simulink model "Strife_Simulation"  (R2020b)
settings: Solver=VariableStepAuto  StartTime=0.0  StopTime=10.0  RelTol=1e-3
libraries: simulink_extras x1, shared3dof x1
settings Model: Creator=bowen  LastModifiedBy=bowen

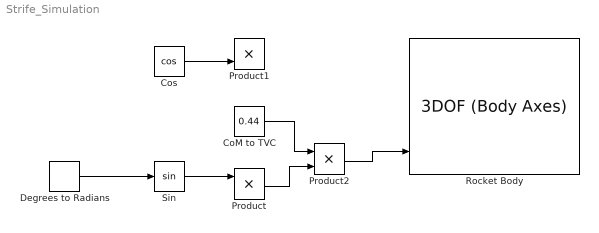
== system Strife_Simulation ==
  CoM to TVC : Constant  Value=0.44
  Cos : Trigonometry  Operator=cos
  Degrees to Radians : simulink_extras/Transformations/Degrees to Radians
  Product : Product
  Product1 : Product
  Product2 : Product
  Rocket Body : shared3dof/3DOF (Body Axes)  units=Metric (MKS)  mtype=Fixed  v_ini=100  theta_ini=0  alpha_ini=0  pos_ini=[0 0]  q_ini=0  mass=1.0  mass_e=0.5  mass_f=3.0  Iyy=1.0  Iyy_e=0.5  Iyy_f=3.0  g_in=Internal  g=9.81  vre_flag=on  abi_flag=off  aMode=0  vel_statename=''  theta_statename=''  pos_statename=''  q_statename=''  mass_statename=''
      settings: SourceProductBaseCode=AE,PW,MT,UV,VE,VP
  Sin : Trigonometry
  wires:
  CoM to TVC/1 -> Product2/1
  Product/1 -> Product2/2
  Product2/1 -> Rocket Body/3
  Sin/1 -> Product/1
  Degrees to Radians/1 -> Sin/1
  Cos/1 -> Product1/2
